simulink model "Nonlinear_model"  (R2015b)
settings: Solver=VariableStepAuto  SolverMode=SingleTasking  StartTime=0.0  StopTime=10.0  RelTol=1e-3
values from neighbouring files (symbols this model uses):
  b = 0.2    [HOMEWORK..m]
  g = 9.81    [HOMEWORK..m]
  M = M_1*1.05+m    (= 11.3)    [HOMEWORK..m]
  m = 1.64    [HOMEWORK..m]
  theta_bar = 0    [HOMEWORK..m]
  theta_bar_dot = 0    [HOMEWORK..m]
  x_bar = 0    [HOMEWORK..m]
  x_bar_dot = 0    [HOMEWORK..m]
undefined symbols (not defined in the file or in its folder): J, L
settings Model: Creator=Sina  LastModifiedBy=Hp
settings DataIOCC: LimitDataPoints=off  ReturnWorkspaceOutputs=on
settings DebuggingCC: AllowSymbolicDim=on  SFUnexpectedBacktrackingDiag=error  SFNoUnconditionalDefaultTransitionDiag=error
settings ModelReferenceCC: PropagateSignalLabelsOutOfModel=on
settings SFSimCC: SimUseLocalCustomCode=on
settings RTWCC: RTWUseLocalCustomCode=on
settings GRTTargetCC: TargetLangStandard=C99 (ISO)
settings ConfigComp: CovMetricSettings=dwe  CovHtmlReporting=off  CovSaveCumulativeToWorkspaceVar=off  CovSaveSingleToWorkspaceVar=off  CovModelRefEnable=Off  CovExternalEMLEnable=on

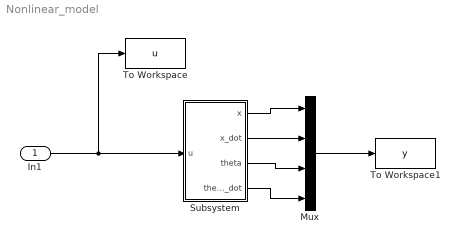
== system Nonlinear_model ==
  In1 : Inport
  Mux : Mux
  Subsystem : Subsystem
  To Workspace : ToWorkspace  VariableName=u  SampleTime=-1
  To Workspace1 : ToWorkspace  VariableName=y  SampleTime=-1
  wires:
  Subsystem/1(x) -> Mux/1
  Subsystem/2(x_dot) -> Mux/2
  Subsystem/4(theta_dot) -> Mux/4
  In1/1 -> To Workspace/1, Subsystem/1(u)
  Subsystem/3(theta) -> Mux/3
  Mux/1 -> To Workspace1/1

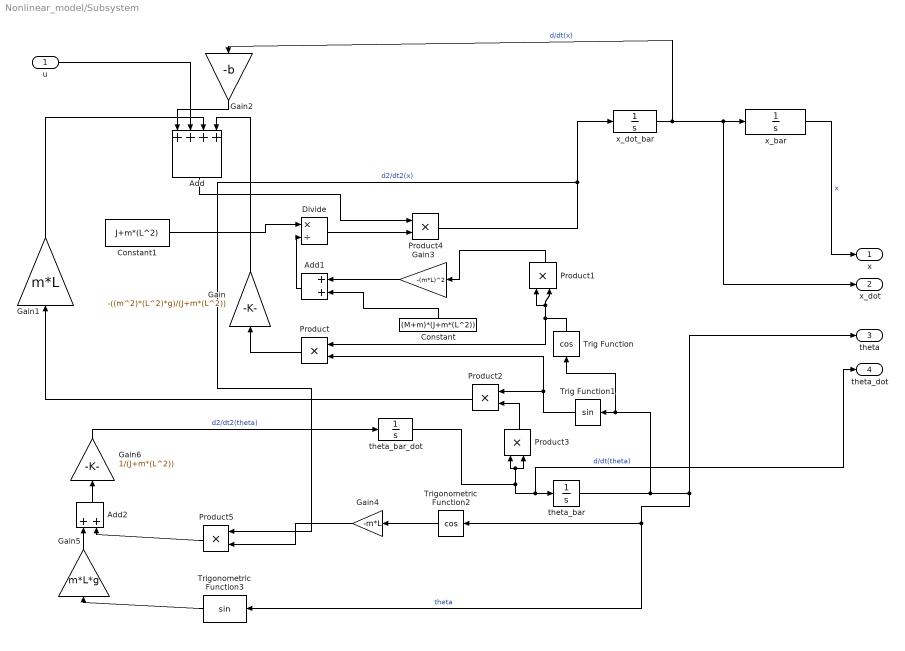
== system Nonlinear_model/Subsystem ==
  u : Inport
  Add : Sum  Inputs=++++
  Add1 : Sum
  Add2 : Sum
  Constant : Constant  Value=(M+m)*(J+m*(L^2))
  Constant1 : Constant  Value=J+m*(L^2)
  Divide : Product  Inputs=*/
  Gain : Gain  Gain=-((m^2)*(L^2)*g)/(J+m*(L^2))
  Gain1 : Gain  Gain=m*L
  Gain2 : Gain  Gain=-b
  Gain3 : Gain  Gain=-(m*L)^2
  Gain4 : Gain  Gain=-m*L
  Gain5 : Gain  Gain=m*L*g
  Gain6 : Gain  Gain=1/(J+m*(L^2))
  Product{,1..5} (6 alike) : Product
  Trig Function : Trigonometry  Operator=cos
  Trig Function1 : Trigonometry
  Trigonometric Function2 : Trigonometry  Operator=cos
  Trigonometric Function3 : Trigonometry
  theta_bar : Integrator  InitialCondition=theta_bar
  theta_bar_dot : Integrator  InitialCondition=theta_bar_dot
  x_bar : Integrator  InitialCondition=x_bar
  x_dot_bar : Integrator  InitialCondition=x_bar_dot
  x : Outport
  x_dot : Outport  Port=2
  theta : Outport  Port=3
  theta_dot : Outport  Port=4
  wires:
  x_dot_bar/1 -> x_dot/1, x_bar/1, Gain2/1  "d/dt(x)"
  Trig Function/1 -> Product/1, Product1/1, Product1/2
  Product4/1 -> x_dot_bar/1, Product5/1  "d2/dt2(x)"
  x_bar/1 -> x/1  "x"
  theta_bar_dot/1 -> theta_dot/1, theta_bar/1, Product3/1, Product3/2  "d/dt(theta)"
  theta_bar/1 -> theta/1, Trigonometric Function3/1, Trigonometric Function2/1, Trig Function/1, Trig Function1/1  "theta"
  Constant/1 -> Add1/2
  Trig Function1/1 -> Product/2, Product2/1
  Product5/1 -> Add2/2
  Product3/1 -> Product2/2
  Trigonometric Function2/1 -> Gain4/1
  Gain1/1 -> Add/3
  Product2/1 -> Gain1/1
  Product/1 -> Gain/1
  Gain2/1 -> Add/1
  Gain5/1 -> Add2/1
  Trigonometric Function3/1 -> Gain5/1
  Add1/1 -> Divide/2
  Gain4/1 -> Product5/2
  Add/1 -> Product4/1
  Divide/1 -> Product4/2
  Gain6/1 -> theta_bar_dot/1  "d2/dt2(theta)"
  Add2/1 -> Gain6/1
  Gain/1 -> Add/4
  Constant1/1 -> Divide/1
  u/1 -> Add/2
  Gain3/1 -> Add1/1
  Product1/1 -> Gain3/1
